simulink model "Ball_Estimation_2_1"  (Simulink 8.0)
settings: Solver=ode4  StartTime=0.0  StopTime=inf  FixedStep=sample_time  RelTol=1e-3
InitFcn:
  | sample_time=0.005;%0.004;%0.0025;%0.02;
  | sample_time_Vicon = 0.005;
  | DeltaT = 0.02;
  | g = 9.81;
  | H0 = g%0.3165;
  | 
  | Q6_mass = 0.95;
  | 
  | Q6_Omega_r = 1.5; %for horizon ref
  | Q6_Zeta_r = 0.7; %for horizon ref
  | Q6_Omega_r_h = 2;%for vertical ref
  | Q6_Zeta_r_h = 1; %for vertical ref
  | 
  | 
  | Q6_Omega = 1.5; %for horizon control
  | Q6_Zeta = 0.7; %for horizon control
  | Q6_Omega_h= 2; %for vertical control
  | Q6_Zeta_h = 0.7; %for vertical control
  | 
  | 
  | Q6_acc_max = 5;%horizontal max acc
  | Q6_acc_max_h = 3;%horizontal max acc
  | 
  | omega_circle = 72*pi/180;
  | omega_h = 0.1;%Ascending speed
  | PI = pi;
  | Circle_R = 2.5;
  | MAX_Height = -2;
undefined symbols (not defined in the file or in its folder): DiscIntNeverNeededParam, PosRefSystem, X330_Control
libraries: simulink x2, dspadpt3 x2
(part 1 of 2)
settings Model: Creator=ttcl3  LastModifiedBy=Vicon
settings SolverCC: MaxConsecutiveMinStep=auto
settings DataIOCC: SignalLoggingSaveFormat=ModelDataLogs
settings DebuggingCC: MultiTaskRateTransMsg=warning  FcnCallInpInsideContextMsg=UseLocalSettings
settings SFSimCC: SimParseCustomCode=off
settings CodeAppCC: CustomSymbolStrType=$N$R$M_T
settings GRTTargetCC: CombineOutputUpdateFcns=off  GRTInterface=on

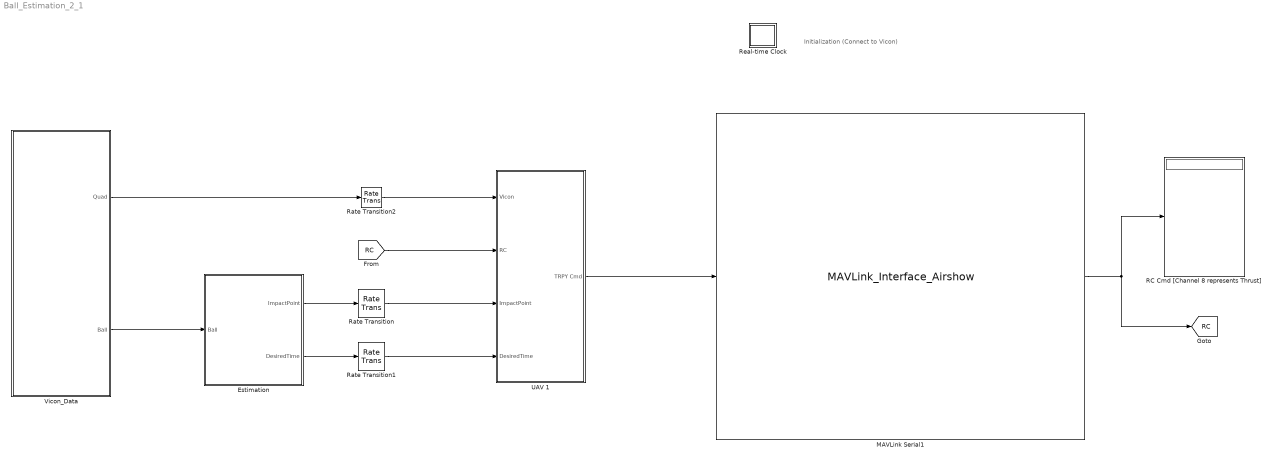
== system Ball_Estimation_2_1 ==
  note: Initialization
      | (Connect to Vicon)
  Estimation : Subsystem
  MAVLink Serial1 : S-Function  FunctionName=MAVLink_Interface_Airshow  Parameters=COM_Port,Baud_Rate,MSG_INPUT,MSG_OUTPUT  EnableBusSupport=off  mask{COM_Port='COM5', Baud_Rate=57600, ATTITUDE_OUT=off, RC_SCALED=on, Quads_1=on, Quads_2=off, Quads_3=off, Quads_4=off, Quads_5=off, Quads_6=off}
      mask prompts: COM_Port "COM Port"; Baud_Rate "Baud Rate"; ATTITUDE_OUT "DEBUG"; RC_SCALED "RC CHANNELS SCALED"; Quads_1 "1 Quad"; Quads_2 "2 Quad"; Quads_3 "3 Quad"; Quads_4 "4 Quad"; Quads_5 "5 Quad"; Quads_6 "6 Quad"
      mask init:
      | MSG_ID_NUM_INPUT = [ uint8(221) uint8(222) uint8(223) uint8(224) uint8(225) uint8(226)];
      | MSG_ID_NAME_INPUT = [Quads_1 Quads_2 Quads_3 Quads_4 Quads_5 Quads_6];
      | 
      | MSG_ID_NUM_OUTPUT = [uint8(34) uint8(30)];
      | MSG_ID_NAME_OUTPUT = [RC_SCALED ATTITUDE_OUT ];
      | 
      | idx_input = find(MSG_ID_NAME_INPUT);
      | MSG_INPUT = MSG_ID_NUM_INPUT(idx_input);
      | 
      | idx_output = find(MSG_ID_NAME_OUTPUT);
      | MSG_OUTPUT = MSG_ID_NUM_OUTPUT(idx_output);
      mask Display:
      | % Block image
      | image(imread('10-inch Quad Heat Map.png'));
      | 
      | %Label block
      | fprintf('MAVLink Serial\n%s\n%dbps', COM_Port,  Baud_Rate)
      | 
      | 
      | %Label input ports
      | 
      | in = 1;
      | if (Quads_1 == 1)
      |     port_label('input', in, 'Quads_1');
      |     in = in + 1;
      | end
      | 
      | if (Quads_2 == 1)
      |     port_label('input', in, 'Quads_2');
      |     in = in + 1;
      | end
      | 
      | if (Quads_3 == 1)
      |     port_label('input', in, 'Quads_3');
      |     in = in + 1;
      | end
      | 
      | if (Quads_4 == 1)
      |     port_label('input', in, 'Quads_4');
      |     in = in + 1;
      | end
      | 
      | if (Quads_5 == 1)
      |     port_label('input', in, 'Quads_5');
      |     in = in + 1;
      | end
      | 
      | 
      | if (Quads_6 == 1)
      |     port_label('input', in, 'Quads_6');
      |     in = in + 1;
      | end
      | %Label output ports
      | 
      | out = 1;
      | if (RC_SCALED == 1)
      |     port_label('output', out, 'RC CMD');
      |     out = out + 1;
      | end
      | 
      | if (ATTITUDE_OUT == 1)
      |     port_label('output', out, 'DEBUG');
      |     out = out + 1;
      | end
  RC Cmd [Channel 8 represents Thrust] : Display
  Rate Transition : RateTransition  OutPortSampleTime=0.02
  Rate Transition1 : RateTransition  OutPortSampleTime=0.02
  Rate Transition2 : RateTransition  OutPortSampleTime=0.02
  Real-time Clock : Subsystem  mask(Real-time Clock){sample_time=0.02, tolerance=1}
      mask prompts: sample_time "Synchronize with real-time every n seconds:"; tolerance "Real-time warning tolerance (seconds):"
      mask help: Real-time Synchronization Block
      mask Help: This block synchronizes simulation time with the PC real-time clock or UNIX system clock. The first dialog entry is the period at which the clock is checked to insure real-time synchronization. The second dialog entry is the number of seconds that the simulation time must be within real-time before a warning is printed.
      mask Display: plot(0,0,100,100,[40,60,60,54,54,64,69,76,82,77,81,83,83,81,78,74,70,64,57,49,41,35,32,30,30,31,34,40,47,47,40,40],[90,90,85,85,80,79,76,87,80,70,64,57,49,41,33,28,24,22,21,23,25,31,37,46,56,65,73,78,80,85,85,90],[69,53,53],[64,50,73])
  UAV 1 : Subsystem
  Vicon_Data : Subsystem
  tag scope: RC=global
  wires:
  Estimation/1(ImpactPoint) -> Rate Transition/1
  Estimation/2(DesiredTime) -> Rate Transition1/1
  [RC] -> UAV 1/2(RC)
  Rate Transition2/1 -> UAV 1/1(Vicon)
  MAVLink Serial1/1 -> [RC], RC Cmd [Channel 8 represents Thrust]/1
  UAV 1/1(TRPY Cmd) -> MAVLink Serial1/1
  Vicon_Data/2(Ball) -> Estimation/1(Ball)
  Vicon_Data/1(Quad) -> Rate Transition2/1
  Rate Transition/1 -> UAV 1/3(ImpactPoint)
  Rate Transition1/1 -> UAV 1/4(DesiredTime)

== system Ball_Estimation_2_1/Estimation ==
  Ball : Inport
  Bus Selector1 : BusSelector  OutputSignals=Position,Velocity
  Trajectory Logic1 : Subsystem
  ImpactPoint : Outport
  DesiredTime : Outport  Port=2
  wires:
  Ball/1 -> Bus Selector1/1
  Bus Selector1/1 -> Trajectory Logic1/1(Ball_Pos)  "<Position>"
  Bus Selector1/2 -> Trajectory Logic1/2(Ball_Vel)  "<Velocity>"
  Trajectory Logic1/1("ImpactPoint ") -> ImpactPoint/1
  Trajectory Logic1/2(DesiredTime) -> DesiredTime/1

== system Ball_Estimation_2_1/Real-time Clock ==
  Real-time Clock : S-Function  FunctionName=rtclock  Parameters=sample_time, tolerance  EnableBusSupport=off

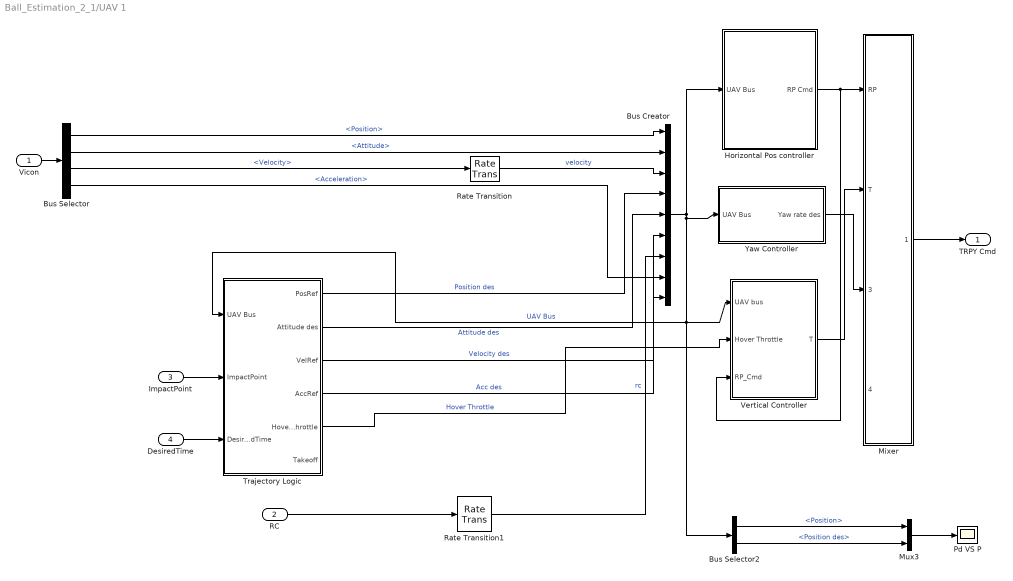
== system Ball_Estimation_2_1/UAV 1 ==
  Vicon : Inport
  RC : Inport  Port=2
  ImpactPoint : Inport  Port=3
  DesiredTime : Inport  Port=4
  Bus Creator : BusCreator  Inputs=9
  Bus Selector : BusSelector  OutputSignals=Position,Attitude,Velocity,Acceleration
  Bus Selector2 : BusSelector  OutputSignals=Position,Position des
  Horizontal Pos controller : Subsystem  AncestorBlock=X330_Control/Horizontal Pos controller  mask{Max_RP=60, Omega=Q6_Omega, PID_i=1, Zeta=Q6_Zeta}
      mask prompts: Max_RP "Cmd Maximum Roll/Pitch (Degree)"; Omega "Omega (P Gain= Omega^2)"; PID_i "I Gain"; Zeta "Zeta (D = 2*Omega*Zeta)"
  Mixer : Subsystem
  Mux3 : Mux  Inputs=2
  Pd VS P : Scope
      settings: TimeRange=19.89708404802744  YMin=-0.75  YMax=0.1
  Rate Transition : RateTransition  OutPortSampleTime=0.02
  Rate Transition1 : RateTransition  OutPortSampleTime=0.02
  Trajectory Logic : Subsystem
  Vertical Controller : Subsystem  AncestorBlock=X330_Control/Vertical Controller  mask{Omega_h=Q6_Omega_h, Zeta_h=Q6_Zeta_h, PID_I_h=1, mass=Q6_mass}
      mask prompts: Omega_h "Omega (P Gain  = Omega^2)"; Zeta_h "Zeta (D Gain = 2*Omega*Zeta)"; PID_I_h "I Gain"
  Yaw Controller : Subsystem  AncestorBlock=X330_Control/Yaw Controller
  TRPY Cmd : Outport
  wires:
  Mux3/1 -> Pd VS P/1
  Bus Selector2/2 -> Mux3/2  "<Position des>"
  Bus Selector2/1 -> Mux3/1  "<Position>"
  Horizontal Pos controller/1(RP Cmd) -> Vertical Controller/3(RP_Cmd), Mixer/1(RP)
  RC/1 -> Rate Transition1/1
  Trajectory Logic/4(AccRef) -> Bus Creator/9  "Acc des"
  Mixer/1(XYZ RPY) -> TRPY Cmd/1
  Vicon/1 -> Bus Selector/1
  Bus Selector/3 -> Rate Transition/1  "<Velocity>"
  Bus Selector/2 -> Bus Creator/2  "<Attitude>"
  Bus Selector/1 -> Bus Creator/1  "<Position>"
  Trajectory Logic/5(HoverThrottle) -> Vertical Controller/2(Hover Throttle)  "Hover Throttle"
  Trajectory Logic/3(VelRef) -> Bus Creator/6  "Velocity des"
  Trajectory Logic/2(Attitude des) -> Bus Creator/5  "Attitude des"
  Trajectory Logic/1(PosRef) -> Bus Creator/4  "Position des"
  Bus Selector/4 -> Bus Creator/8  "<Acceleration>"
  Vertical Controller/1(T) -> Mixer/2(T)
  Yaw Controller/1(Yaw rate des) -> Mixer/3(Yaw rate)
  Bus Creator/1 -> Yaw Controller/1(UAV Bus), Bus Selector2/1, Vertical Controller/1(UAV bus), Trajectory Logic/1(UAV Bus), Horizontal Pos controller/1(UAV Bus)  "UAV Bus"
  Rate Transition1/1 -> Bus Creator/7  "rc"
  Rate Transition/1 -> Bus Creator/3  "velocity"
  ImpactPoint/1 -> Trajectory Logic/2(ImpactPoint)
  DesiredTime/1 -> Trajectory Logic/3(DesiredTime)

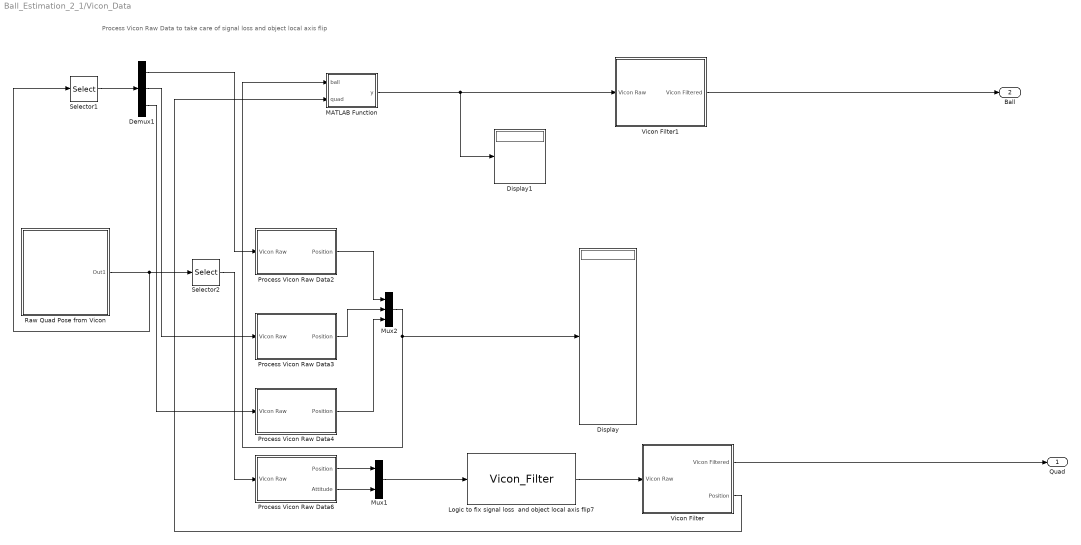
== system Ball_Estimation_2_1/Vicon_Data ==
  note: Process Vicon Raw Data to take care of signal loss and object local axis flip
  Demux1 : Demux  Outputs=3
  Display : Display
  Display1 : Display
  Logic to fix signal loss  and object local axis flip7 : M-S-Function  FunctionName=Vicon_Filter
  MATLAB Function : MATLAB Function  TreatAsAtomicUnit=on
      settings: PermitHierarchicalResolution=ParametersOnly
  Mux1 : Mux  Inputs=2
  Mux2 : Mux  Inputs=3
  Process Vicon Raw Data2 : Subsystem
  Process Vicon Raw Data3 : Subsystem
  Process Vicon Raw Data4 : Subsystem
  Process Vicon Raw Data6 : Subsystem
  Raw Quad Pose from Vicon : Subsystem
  Selector1 : Selector  InputPortWidth=18  IndexOptions=Index vector (dialog)  Indices=[10 11 12 13 14 15 16 17 18]  OutputSizes=1
  Selector2 : Selector  InputPortWidth=18  IndexOptions=Index vector (dialog)  Indices=[1 2 3 4 5 6]  OutputSizes=1
  Vicon Filter : Subsystem  AncestorBlock=X330_Control/Vicon Filter
  Vicon Filter1 : Subsystem  AncestorBlock=X330_Control/Vicon Filter
  Quad : Outport
  Ball : Outport  Port=2
  wires:
  Raw Quad Pose from Vicon/1(Out1) -> Selector1/1, Selector2/1
  Selector2/1 -> Process Vicon Raw Data6/1(Vicon Raw)
  Logic to fix signal loss  and object local axis flip7/1 -> Vicon Filter/1(Vicon Raw)
  Process Vicon Raw Data6/1(Position) -> Mux1/1
  Process Vicon Raw Data6/2(Attitude) -> Mux1/2
  Mux1/1 -> Logic to fix signal loss  and object local axis flip7/1
  Vicon Filter/1(Vicon Filtered) -> Quad/1
  Vicon Filter/2(Position) -> MATLAB Function/2(quad)
  Selector1/1 -> Demux1/1
  Demux1/1 -> Process Vicon Raw Data2/1(Vicon Raw)
  Demux1/2 -> Process Vicon Raw Data3/1(Vicon Raw)
  Demux1/3 -> Process Vicon Raw Data4/1(Vicon Raw)
  Process Vicon Raw Data2/1(Position) -> Mux2/1
  Process Vicon Raw Data3/1(Position) -> Mux2/2
  Process Vicon Raw Data4/1(Position) -> Mux2/3
  Mux2/1 -> MATLAB Function/1(ball), Display/1
  MATLAB Function/1(y) -> Display1/1, Vicon Filter1/1(Vicon Raw)
  Vicon Filter1/1(Vicon Filtered) -> Ball/1

== system Ball_Estimation_2_1/Estimation/Trajectory Logic1 ==
  Ball_Pos : Inport
  Ball_Vel : Inport  Port=2
  Ball pos : Scope
      settings: YMin=-4  YMax=0  SaveName=ScopeData4  MaxDataPoints=50000
  UAV SF : Stateflow chart  TreatAsAtomicUnit=on
      settings: PermitHierarchicalResolution=ParametersOnly
  "ImpactPoint " : Outport
  DesiredTime : Outport  Port=2
  wires:
  Ball_Pos/1 -> Ball pos/1, UAV SF/1(Sc_Pos)
  Ball_Vel/1 -> UAV SF/2(Sc_Vel)
  UAV SF/1(ImpactPoint) -> "ImpactPoint "/1
  UAV SF/2(DesiredTime) -> DesiredTime/1

== system Ball_Estimation_2_1/UAV 1/Horizontal Pos controller ==
  UAV Bus : Inport
  Horizontal Position Controller : Subsystem
  RP Cmd : Outport
  wires:
  Horizontal Position Controller/1(RP Cmd (Radian)) -> RP Cmd/1
  UAV Bus/1 -> Horizontal Position Controller/1(UAV Bus)

== system Ball_Estimation_2_1/UAV 1/Mixer ==
  note: 7x1 vector (usec, XYZRPY)
  RP : Inport
  T : Inport  Port=2
  Yaw rate : Inport  Port=3
  PWM : Inport  Port=4
  Gain : Gain  Gain=180/pi
  Mode : Constant  SampleTime=0.02
  Mux1 : Mux  Inputs=5
  "[-1, 1]" : Fcn  Expr=u(1)*2-1
  XYZ RPY : Outport
  wires:
  "[-1, 1]"/1 -> Mux1/1
  Gain/1 -> Mux1/2
  PWM/1 -> Mux1/5
  Mode/1 -> Mux1/4
  Yaw rate/1 -> Mux1/3
  RP/1 -> Gain/1
  T/1 -> "[-1, 1]"/1
  Mux1/1 -> XYZ RPY/1

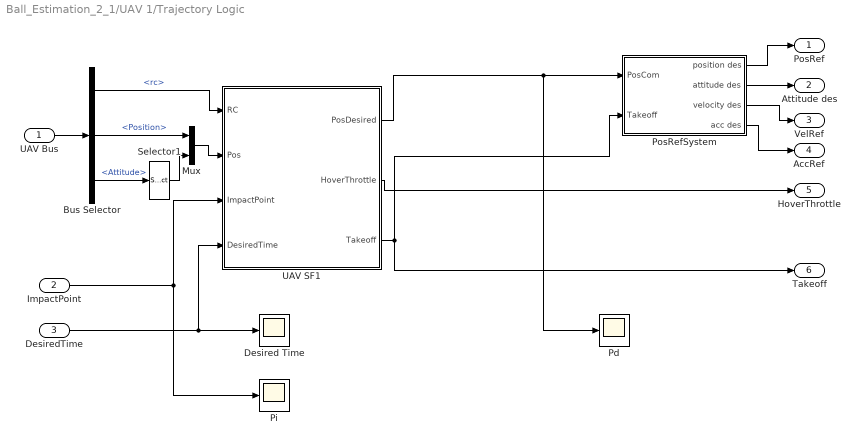
== system Ball_Estimation_2_1/UAV 1/Trajectory Logic ==
  UAV Bus : Inport
  ImpactPoint : Inport  Port=2
  DesiredTime : Inport  Port=3
  Bus Selector : BusSelector  OutputSignals=rc,Position,Attitude
  Desired Time : Scope
      settings: YMin=-0.01  YMax=0.17  SaveName=ScopeData6  MaxDataPoints=500000
  Mux : Mux  Inputs=2
  Pd : Scope
  Pi : Scope
      settings: TimeRange=4.304464104457637  YMin=-0.9662149265126931  YMax=0.8352739072342059  SaveName=ScopeData2
  PosRefSystem : Subsystem  AncestorBlock=X330_Control/PosRefSystem  mask{Omega_r=Q6_Omega_r, Zeta_r=Q6_Zeta_r, Acc_Max=Q6_acc_max, Omega_h_r=Q6_Omega_r_h, Zeta_h_r=Q6_Zeta_r_h, Acc_h_Max=Q6_acc_max_h}
      mask prompts: Omega_r "Omega_r (P Gain= Omega_r^2)"; Zeta_r "Zeta_r (D = 2*Omega_r*Zeta_r)"
  Selector1 : Selector  InputPortWidth=3  IndexOptions=Index vector (dialog)  Indices=[3]  OutputSizes=1
  UAV SF1 : Stateflow chart  TreatAsAtomicUnit=on
      settings: PermitHierarchicalResolution=ParametersOnly
  PosRef : Outport
  Attitude des : Outport  Port=2
  VelRef : Outport  Port=3
  AccRef : Outport  Port=4
  HoverThrottle : Outport  Port=5
  Takeoff : Outport  Port=6
  wires:
  PosRefSystem/2(attitude des) -> Attitude des/1
  PosRefSystem/4(acc des) -> AccRef/1
  PosRefSystem/3(velocity des) -> VelRef/1
  PosRefSystem/1(position des) -> PosRef/1
  Mux/1 -> UAV SF1/2(Pos)
  Selector1/1 -> Mux/2
  Bus Selector/3 -> Selector1/1  "<Attitude>"
  Bus Selector/2 -> Mux/1  "<Position>"
  UAV Bus/1 -> Bus Selector/1
  ImpactPoint/1 -> Pi/1, UAV SF1/3(ImpactPoint)
  UAV SF1/2(HoverThrottle) -> HoverThrottle/1
  Bus Selector/1 -> UAV SF1/1(RC)  "<rc>"
  UAV SF1/3(Takeoff) -> Takeoff/1, PosRefSystem/2(Takeoff)
  DesiredTime/1 -> Desired Time/1, UAV SF1/4(DesiredTime)
  UAV SF1/1(PosDesired) -> Pd/1, PosRefSystem/1(PosCom)

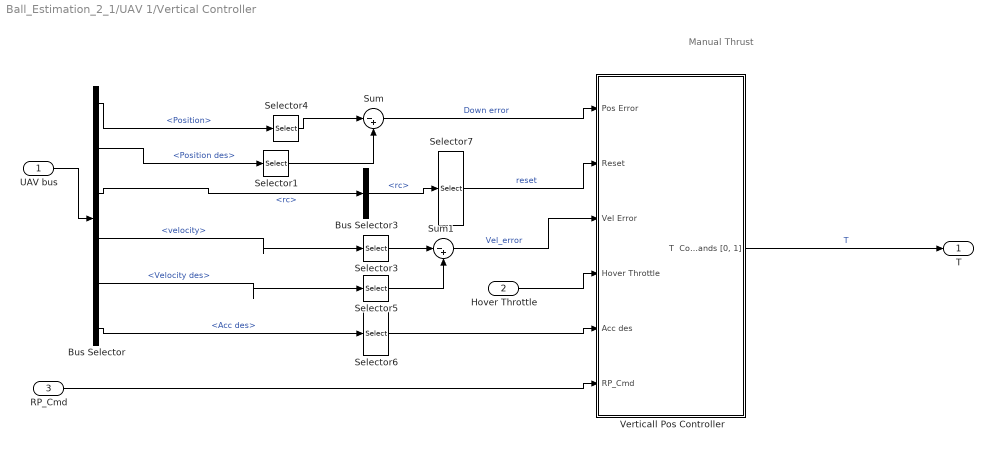
== system Ball_Estimation_2_1/UAV 1/Vertical Controller ==
  note: Manual Thrust
  UAV bus : Inport
  Hover Throttle : Inport  Port=2
  RP_Cmd : Inport  Port=3
  Bus Selector : BusSelector  OutputSignals=Position,Position des,rc,velocity,Velocity des,Acc des
  Bus Selector3 : BusSelector  OutputSignals=rc
  Selector{1,3..5} (4 alike) : Selector  InputPortWidth=3  IndexOptions=Index vector (dialog)  Indices=[3]  OutputSizes=1
  Selector6 : Selector  InputPortWidth=4  IndexOptions=Index vector (dialog)  Indices=[3]  OutputSizes=1
  Selector7 : Selector  InputPortWidth=8  IndexOptions=Index vector (dialog)  Indices=[5]  OutputSizes=1
  Sum : Sum  Inputs=|-+
  Sum1 : Sum  Inputs=|-+
  Verticall Pos Controller : Subsystem
  T : Outport
  wires:
  RP_Cmd/1 -> Verticall Pos Controller/6(RP_Cmd)
  Verticall Pos Controller/1("T  Commands [0, 1]") -> T/1  "T"
  Selector6/1 -> Verticall Pos Controller/5(Acc des)
  Bus Selector/6 -> Selector6/1  "<Acc des>"
  Hover Throttle/1 -> Verticall Pos Controller/4(Hover Throttle)
  Bus Selector/5 -> Selector5/1  "<Velocity des>"
  Bus Selector/4 -> Selector3/1  "<velocity>"
  Selector5/1 -> Sum1/2
  Selector3/1 -> Sum1/1
  Sum1/1 -> Verticall Pos Controller/3(Vel Error)  "Vel_error"
  Selector7/1 -> Verticall Pos Controller/2(Reset)  "reset"
  Bus Selector3/1 -> Selector7/1  "<rc>"
  Selector1/1 -> Sum/2
  Selector4/1 -> Sum/1
  Sum/1 -> Verticall Pos Controller/1(Pos Error)  "Down error"
  Bus Selector/2 -> Selector1/1  "<Position des>"
  Bus Selector/1 -> Selector4/1  "<Position>"
  Bus Selector/3 -> Bus Selector3/1  "<rc>"
  UAV bus/1 -> Bus Selector/1

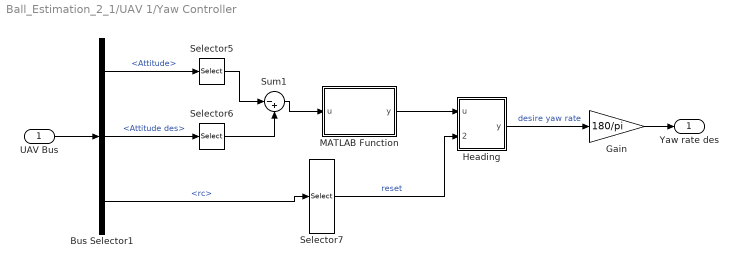
== system Ball_Estimation_2_1/UAV 1/Yaw Controller ==
  UAV Bus : Inport
  Bus Selector1 : BusSelector  OutputSignals=Attitude,Attitude des,rc
  Gain : Gain  Gain=180/pi
  Heading : Subsystem  AncestorBlock=simulink/Continuous/PID Controller  DialogController=pidpack.PIDConfig.pidDDGCreate  DialogControllerArgs=DataTag0  mask(PID 1dof){Controller=PI, TimeDomain=Discrete-time, SampleTime=0.02, IntegratorMethod=Trapezoidal, FilterMethod=Trapezoidal, Form=Parallel, P=3, I=1, D=0, N=100, InitialConditionSource=internal, InitialConditionForIntegrator=0, InitialConditionForFilter=0, ExternalReset=rising, IgnoreLimit=off, ZeroCross=on, LimitOutput=on, UpperSaturationLimit=300*pi/180, LowerSaturationLimit=-300*pi/180, LinearizeAsGain=off, AntiWindupMode=none, Kb=1, TrackingMode=off, Kt=1, RndMeth=Floor, SaturateOnIntegerOverflow=off, LockScale=off, PParamMin=[], PParamMax=[], PParamDataTypeStr=Inherit: Inherit via internal rule, IParamMin=[], IParamMax=[], IParamDataTypeStr=Inherit: Inherit via internal rule, DParamMin=[], DParamMax=[], DParamDataTypeStr=Inherit: Inherit via internal rule, NParamMin=[], NParamMax=[], NParamDataTypeStr=Inherit: Inherit via internal rule, KbParamMin=[], KbParamMax=[], KbParamDataTypeStr=Inherit: Inherit via internal rule, KtParamMin=[], KtParamMax=[], KtParamDataTypeStr=Inherit: Inherit via internal rule, POutMin=[], POutMax=[], POutDataTypeStr=Inherit: Inherit via internal rule, IOutMin=[], IOutMax=[], IOutDataTypeStr=Inherit: Inherit via internal rule, DOutMin=[], DOutMax=[], DOutDataTypeStr=Inherit: Inherit via internal rule, NOutMin=[], NOutMax=[], NOutDataTypeStr=Inherit: Inherit via internal rule, KbOutMin=[], KbOutMax=[], KbOutDataTypeStr=Inherit: Inherit via internal rule, KtOutMin=[], KtOutMax=[], KtOutDataTypeStr=Inherit: Inherit via internal rule, IntegratorOutMin=[], IntegratorOutMax=[], IntegratorOutDataTypeStr=Inherit: Inherit via internal rule, FilterOutMin=[], FilterOutMax=[], FilterOutDataTypeStr=Inherit: Inherit via internal rule, SumOutMin=[], SumOutMax=[], SumOutDataTypeStr=Inherit: Inherit via internal rule, SumI1OutMin=[], SumI1OutMax=[], SumI1OutDataTypeStr=Inherit: Inherit via internal rule, SumI2OutMin=[], SumI2OutMax=[], SumI2OutDataTypeStr=Inherit: Inherit via internal rule, SumI3OutMin=[], SumI3OutMax=[], SumI3OutDataTypeStr=Inherit: Inherit via internal rule, SumDOutMin=[], SumDOutMax=[], SumDOutDataTypeStr=Inherit: Inherit via internal rule, SumAccumDataTypeStr=Inherit: Inherit via internal rule, SumI1AccumDataTypeStr=Inherit: Inherit via internal rule, SumI2AccumDataTypeStr=Inherit: Inherit via internal rule, SumI3AccumDataTypeStr=Inherit: Inherit via internal rule, SumDAccumDataTypeStr=Inherit: Inherit via internal rule, SaturationOutMin=[], SaturationOutMax=[], SaturationOutDataTypeStr=Inherit: Same as input, IntegratorContinuousStateAttributes='', IntegratorStateIdentifier=, IntegratorStateMustResolveToSignalObject=off, IntegratorRTWStateStorageClass=Auto, IntegratorRTWStateStorageTypeQualifier=, FilterContinuousStateAttributes='', FilterStateIdentifier=, FilterStateMustResolveToSignalObject=off, FilterRTWStateStorageClass=Auto, FilterRTWStateStorageTypeQualifier=}
      mask prompts: TimeDomain "Time domain:"; SampleTime "Sample time (-1 for inherited):"; IntegratorMethod "Integrator method:"; FilterMethod "Filter method:"; P "Proportional (P):"; I "Integral (I):"; D "Derivative (D):"; N "Filter coefficient (N):"; InitialConditionSource "Source:"; InitialConditionForIntegrator "Integrator:"; InitialConditionForFilter "Filter:"; ExternalReset "External reset:"; IgnoreLimit "Ignore reset when linearizing"; ZeroCross "Enable zero-crossing detection"; LimitOutput "Limit output"; UpperSaturationLimit "Upper saturation limit:"; LowerSaturationLimit "Lower saturation limit:"; LinearizeAsGain "Ignore saturation when linearizing"; AntiWindupMode "Anti-windup method:"; Kb "Back-calculation coefficient (Kb):"; TrackingMode "Enable tracking mode"; Kt "Tracking coefficient (Kt):"; RndMeth "Integer rounding mode:"; SaturateOnIntegerOverflow "Saturate on integer overflow"; LockScale "Lock data type settings against changes by the fixed-point tools"; PParamMin "P parameter minimum:"; PParamMax "P parameter maximum:"; PParamDataTypeStr "P parameter:"; IParamMin "I parameter minimum:"; IParamMax "I parameter maximum:"; IParamDataTypeStr "I parameter:"; DParamMin "D parameter minimum:"; DParamMax "D parameter maximum:"; DParamDataTypeStr "D parameter:"; NParamMin "N parameter minimum:"; NParamMax "N parameter maximum:"; NParamDataTypeStr "N parameter:"; KbParamMin "Kb parameter minimum:"; KbParamMax "Kb parameter maximum:"; KbParamDataTypeStr "Kb parameter:"; KtParamMin "Kt parameter minimum:"; KtParamMax "Kt parameter maximum:"; KtParamDataTypeStr "Kt parameter:"; POutMin "P product output minimum:"; POutMax "P product output maximum:"; POutDataTypeStr "P product output:"; IOutMin "I product output minimum:"; IOutMax "I product output maximum:"; IOutDataTypeStr "I product output:"; DOutMin "D product output minimum:"; DOutMax "D product output maximum:"; DOutDataTypeStr "D product output:"; NOutMin "N product output minimum:"; NOutMax "N product output maximum:"; NOutDataTypeStr "N product output:"; KbOutMin "Kb product output minimum:"; KbOutMax "Kb product output maximum:"; KbOutDataTypeStr "Kb product output:"; KtOutMin "Kt product output minimum:"; KtOutMax "Kt product output maximum:"; KtOutDataTypeStr "Kt product output:"; IntegratorOutMin "Integrator output minimum:"; IntegratorOutMax "Integrator output maximum:"; IntegratorOutDataTypeStr "Integrator output:"; FilterOutMin "Filter output minimum:"; FilterOutMax "Filter output maximum:"; FilterOutDataTypeStr "Filter output:"; SumOutMin "Sum output minimum:"; SumOutMax "Sum output maximum:"; SumOutDataTypeStr "Sum output:"; SumI1OutMin "SumI1 output minimum:"; SumI1OutMax "SumI1 output maximum:"; SumI1OutDataTypeStr "SumI1 output:"; SumI2OutMin "SumI2 output minimum:"; SumI2OutMax "SumI2 output maximum:"; SumI2OutDataTypeStr "SumI2 output:"; SumI3OutMin "SumI3 output minimum:"; SumI3OutMax "SumI3 output maximum:"; SumI3OutDataTypeStr "SumI3 output:"; SumDOutMin "SumD output minimum:"; SumDOutMax "SumD output maximum:"; SumDOutDataTypeStr "SumD output:"; SumAccumDataTypeStr "Accumulator of Sum:"; SumI1AccumDataTypeStr "Accumulator of SumI1:"; SumI2AccumDataTypeStr "Accumulator of SumI2:"; SumI3AccumDataTypeStr "Accumulator of SumI3:"; SumDAccumDataTypeStr "Accumulator of SumD:"; SaturationOutMin "Saturation output minimum:"; SaturationOutMax "Saturation output maximum:"; SaturationOutDataTypeStr "Saturation output:"; IntegratorContinuousStateAttributes "State name: (e.g., 'position')"; IntegratorStateIdentifier "State name:"; IntegratorStateMustResolveToSignalObject "State name must resolve to Simulink signal object"; IntegratorRTWStateStorageClass "Code generation storage class:"; IntegratorRTWStateStorageTypeQualifier "Code generation storage type qualifier:"; FilterContinuousStateAttributes "State name: (e.g., 'position')"; FilterStateIdentifier "State name:"; FilterStateMustResolveToSignalObject "State name must resolve to Simulink signal object"; FilterRTWStateStorageClass "Code generation storage class:"; FilterRTWStateStorageTypeQualifier "Code generation storage type qualifier:"
      mask help: This block implements continuous- and discrete-time PID control algorithms and includes advanced features such as anti-windup, external reset, and signal tracking. You can tune the PID gains automatically using the 'Tune...' button (requires Simulink Control Design).
      mask init:
      | pidpack.PIDConfig.configPID(gcbh);
      settings: DeleteFcn=pidpack.PIDConfig.closeTuner(gcbh)  ModelCloseFcn=pidpack.PIDConfig.closeTuner(gcbh)  NameChangeFcn=pidpack.PIDConfig.updateTunerName(gcbh)
      mask TypeOptions Controller: PID | PI | PD | P | I
      mask TypeOptions TimeDomain: Continuous-time | Discrete-time
      mask TypeOptions IntegratorMethod: Forward Euler | Backward Euler | Trapezoidal
      mask TypeOptions FilterMethod: Forward Euler | Backward Euler | Trapezoidal
      mask TypeOptions Form: Ideal | Parallel
      mask TypeOptions InitialConditionSource: internal | external
      mask TypeOptions ExternalReset: none | rising | falling | either | level
      mask TypeOptions AntiWindupMode: none | back-calculation | clamping
      mask TypeOptions RndMeth: Ceiling | Convergent | Floor | Nearest | Round | Simplest | Zero
      mask TypeOptions IntegratorRTWStateStorageClass: Auto | ExportedGlobal | ImportedExtern | ImportedExternPointer
      mask TypeOptions FilterRTWStateStorageClass: Auto | ExportedGlobal | ImportedExtern | ImportedExternPointer
      mask Display:
      | image(imread(fullfile(matlabroot,'toolbox','simulink','blocks','@pidpack','@PIDMasks','images','blank.png'),'png'),[0 0 1 1]);
      | disp('PI(z)')
      | port_label('input',1, '');
      | port_label('output',1, '');
      | plot([0 4 4 7]+2,[0 0 8 8]+8);
      | plot([1 4 6]+2,[3 6 3]+8);
      | plot([0 4 6 10]+32,[0 0 8 8]+18);
  MATLAB Function : MATLAB Function  TreatAsAtomicUnit=on
      settings: PermitHierarchicalResolution=ParametersOnly
  Selector5 : Selector  InputPortWidth=3  IndexOptions=Index vector (dialog)  Indices=[3]  OutputSizes=1
  Selector6 : Selector  InputPortWidth=3  IndexOptions=Index vector (dialog)  Indices=[3]  OutputSizes=1
  Selector7 : Selector  InputPortWidth=8  IndexOptions=Index vector (dialog)  Indices=[5]  OutputSizes=1
  Sum1 : Sum  Inputs=|-+
  Yaw rate des : Outport
  wires:
  Bus Selector1/3 -> Selector7/1  "<rc>"
  Bus Selector1/2 -> Selector6/1  "<Attitude des>"
  Selector6/1 -> Sum1/2
  Sum1/1 -> MATLAB Function/1(u)
  MATLAB Function/1(y) -> Heading/1(u)
  UAV Bus/1 -> Bus Selector1/1
  Bus Selector1/1 -> Selector5/1  "<Attitude>"
  Heading/1(y) -> Gain/1  "desire yaw rate"
  Selector7/1 -> Heading/2(RESET)  "reset"
  Selector5/1 -> Sum1/1
  Gain/1 -> Yaw rate des/1

== system Ball_Estimation_2_1/Vicon_Data/Process Vicon Raw Data2 ==
  note: X
  note: Y
  note: Z
  Vicon Raw : Inport
  Demux : Demux  Outputs=3
  Gain1 : Gain  Gain=0.001
  Gain6 : Gain  Gain=-0.001
  Gain7 : Gain  Gain=-0.001
  Matrix Concatenate13 : Concatenate  NumInputs=3  Mode=Multidimensional array
  Position : Outport
  wires:
  Gain1/1 -> Matrix Concatenate13/1
  Demux/1 -> Gain1/1
  Demux/2 -> Gain6/1
  Demux/3 -> Gain7/1
  Gain6/1 -> Matrix Concatenate13/2
  Gain7/1 -> Matrix Concatenate13/3
  Matrix Concatenate13/1 -> Position/1
  Vicon Raw/1 -> Demux/1

== system Ball_Estimation_2_1/Vicon_Data/Process Vicon Raw Data3 ==
  note: Z
  note: Y
  note: X
  Vicon Raw : Inport
  Demux : Demux  Outputs=3
  Gain1 : Gain  Gain=0.001
  Gain6 : Gain  Gain=-0.001
  Gain7 : Gain  Gain=-0.001
  Matrix Concatenate13 : Concatenate  NumInputs=3  Mode=Multidimensional array
  Position : Outport
  wires:
  Vicon Raw/1 -> Demux/1
  Matrix Concatenate13/1 -> Position/1
  Gain7/1 -> Matrix Concatenate13/3
  Gain6/1 -> Matrix Concatenate13/2
  Demux/3 -> Gain7/1
  Demux/2 -> Gain6/1
  Demux/1 -> Gain1/1
  Gain1/1 -> Matrix Concatenate13/1

== system Ball_Estimation_2_1/Vicon_Data/Process Vicon Raw Data4 ==
  note: X
  note: Y
  note: Z
  Vicon Raw : Inport
  Demux : Demux  Outputs=3
  Gain1 : Gain  Gain=0.001
  Gain6 : Gain  Gain=-0.001
  Gain7 : Gain  Gain=-0.001
  Matrix Concatenate13 : Concatenate  NumInputs=3  Mode=Multidimensional array
  Position : Outport
  wires:
  Gain1/1 -> Matrix Concatenate13/1
  Demux/1 -> Gain1/1
  Demux/2 -> Gain6/1
  Demux/3 -> Gain7/1
  Gain6/1 -> Matrix Concatenate13/2
  Gain7/1 -> Matrix Concatenate13/3
  Matrix Concatenate13/1 -> Position/1
  Vicon Raw/1 -> Demux/1

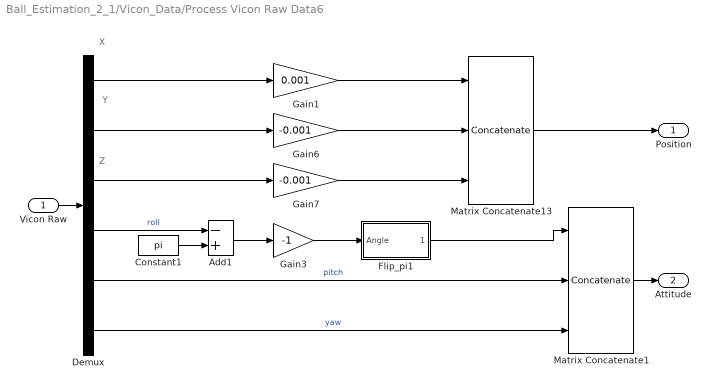
== system Ball_Estimation_2_1/Vicon_Data/Process Vicon Raw Data6 ==
  note: X
  note: Y
  note: Z
  Vicon Raw : Inport
  Add1 : Sum  Inputs=-+
  Constant1 : Constant  Value=pi  OutDataTypeStr=double
  Demux : Demux  Outputs=6
  Flip_pi1 : Subsystem  mask(Flip -pi to pi){}
      mask help: Flips the inputs into the range -pi to pi
      mask Help: Flips the inputs into the range -pi to pi
      mask Display: disp('Flip_pi')
  Gain1 : Gain  Gain=0.001
  Gain3 : Gain  Gain=-1
  Gain6 : Gain  Gain=-0.001
  Gain7 : Gain  Gain=-0.001
  Matrix Concatenate1 : Concatenate  NumInputs=3  Mode=Multidimensional array
  Matrix Concatenate13 : Concatenate  NumInputs=3  Mode=Multidimensional array
  Position : Outport
  Attitude : Outport  Port=2
  wires:
  Constant1/1 -> Add1/2
  Demux/6 -> Matrix Concatenate1/3  "yaw"
  Gain1/1 -> Matrix Concatenate13/1
  Demux/1 -> Gain1/1
  Demux/2 -> Gain6/1
  Demux/3 -> Gain7/1
  Demux/4 -> Add1/1  "roll"
  Gain6/1 -> Matrix Concatenate13/2
  Gain7/1 -> Matrix Concatenate13/3
  Add1/1 -> Gain3/1
  Gain3/1 -> Flip_pi1/1(Angle)
  Demux/5 -> Matrix Concatenate1/2  "pitch"
  Flip_pi1/1(Angle_Flip) -> Matrix Concatenate1/1
  Matrix Concatenate13/1 -> Position/1
  Vicon Raw/1 -> Demux/1
  Matrix Concatenate1/1 -> Attitude/1

== system Ball_Estimation_2_1/Vicon_Data/Raw Quad Pose from Vicon ==
  Constant : Constant
  Interpreted MATLAB Function : MATLABFcn  MATLABFcn=GetViconPose_BallCatching  OutputDimensions=18  SampleTime=0.005
  Out1 : Outport
  wires:
  Constant/1 -> Interpreted MATLAB Function/1
  Interpreted MATLAB Function/1 -> Out1/1

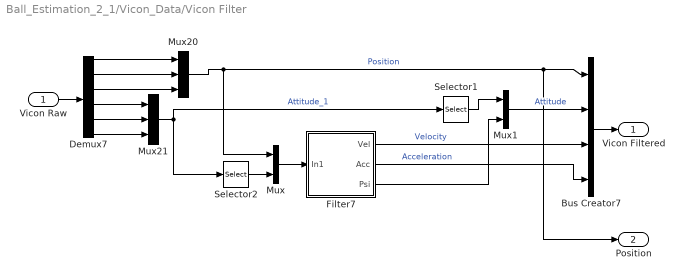
== system Ball_Estimation_2_1/Vicon_Data/Vicon Filter ==
  Vicon Raw : Inport
  Bus Creator7 : BusCreator
  Demux7 : Demux  Outputs=6
  Filter7 : Subsystem
  Mux : Mux  Inputs=2
  Mux1 : Mux  Inputs=2
  Mux20 : Mux  Inputs=3
  Mux21 : Mux  Inputs=3
  Selector1 : Selector  InputPortWidth=3  IndexOptions=Index vector (dialog)  Indices=[1 2]  OutputSizes=1
  Selector2 : Selector  InputPortWidth=3  IndexOptions=Index vector (dialog)  Indices=[3]  OutputSizes=1
  Vicon Filtered : Outport
  Position : Outport  Port=2
  wires:
  Bus Creator7/1 -> Vicon Filtered/1
  Vicon Raw/1 -> Demux7/1
  Mux1/1 -> Bus Creator7/2  "Attitude"
  Selector1/1 -> Mux1/1
  Filter7/3(Psi) -> Mux1/2
  Mux/1 -> Filter7/1(In1)
  Selector2/1 -> Mux/2
  Filter7/2(Acc) -> Bus Creator7/4  "Acceleration"
  Filter7/1(Vel) -> Bus Creator7/3  "Velocity"
  Mux21/1 -> Selector1/1, Selector2/1  "Attitude_1"
  Mux20/1 -> Mux/1, Position/1, Bus Creator7/1  "Position"
  Demux7/2 -> Mux20/2
  Demux7/1 -> Mux20/1
  Demux7/6 -> Mux21/3
  Demux7/5 -> Mux21/2
  Demux7/4 -> Mux21/1
  Demux7/3 -> Mux20/3

== system Ball_Estimation_2_1/Vicon_Data/Vicon Filter1 ==
  Vicon Raw : Inport
  Bus Creator7 : BusCreator  Inputs=3
  Demux7 : Demux  Outputs=6
  Filter7 : Subsystem
  Mux : Mux  Inputs=2
  Mux20 : Mux  Inputs=3
  Mux21 : Mux  Inputs=3
  Selector2 : Selector  InputPortWidth=3  IndexOptions=Index vector (dialog)  Indices=[3]  OutputSizes=1
  Vicon Filtered : Outport
  wires:
  Demux7/3 -> Mux20/3
  Demux7/4 -> Mux21/1
  Demux7/5 -> Mux21/2
  Demux7/6 -> Mux21/3
  Demux7/1 -> Mux20/1
  Demux7/2 -> Mux20/2
  Mux20/1 -> Bus Creator7/1, Mux/1  "Position"
  Mux21/1 -> Selector2/1  "Attitude_1"
  Filter7/1(Vel) -> Bus Creator7/2  "Velocity"
  Filter7/2(Acc) -> Bus Creator7/3  "Acceleration"
  Selector2/1 -> Mux/2
  Mux/1 -> Filter7/1(In1)
  Vicon Raw/1 -> Demux7/1
  Bus Creator7/1 -> Vicon Filtered/1

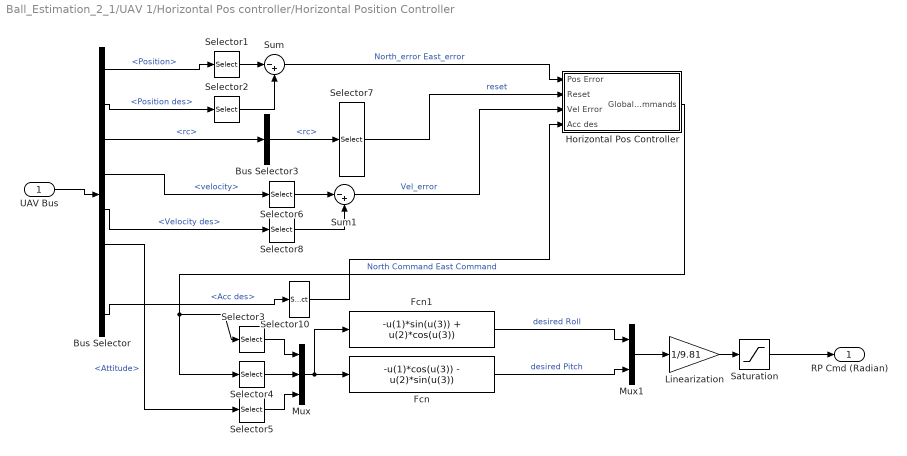
== system Ball_Estimation_2_1/UAV 1/Horizontal Pos controller/Horizontal Position Controller ==
  UAV Bus : Inport
  Bus Selector : BusSelector  OutputSignals=Position,Position des,rc,velocity,Velocity des,Attitude,Acceleration,Acc des
  Bus Selector3 : BusSelector  OutputSignals=rc
  Fcn : Fcn  Expr=-u(1)*cos(u(3)) - u(2)*sin(u(3))
  Fcn1 : Fcn  Expr=-u(1)*sin(u(3)) + u(2)*cos(u(3))
  Horizontal Pos Controller : Subsystem
  Linearization : Gain  Gain=1/9.81  OutDataTypeStr=double
  Mux : Mux  Inputs=3
  Mux1 : Mux  Inputs=2
  Saturation : Saturate  UpperLimit=Max_RP  LowerLimit=-Max_RP
  Selector{1..2,6,8} (4 alike) : Selector  InputPortWidth=3  IndexOptions=Index vector (dialog)  Indices=[1 2]  OutputSizes=1
  Selector10 : Selector  InputPortWidth=4  IndexOptions=Index vector (dialog)  Indices=[1 2]  OutputSizes=1
  Selector3 : Selector  InputPortWidth=2  IndexOptions=Index vector (dialog)  Indices=[1]  OutputSizes=1
  Selector4 : Selector  InputPortWidth=2  IndexOptions=Index vector (dialog)  Indices=[2]  OutputSizes=1
  Selector5 : Selector  InputPortWidth=3  IndexOptions=Index vector (dialog)  Indices=[3]  OutputSizes=1
  Selector7 : Selector  InputPortWidth=8  IndexOptions=Index vector (dialog)  Indices=[5]  OutputSizes=1
  Sum : Sum  Inputs=|-+
  Sum1 : Sum  Inputs=|-+
  RP Cmd (Radian) : Outport
  wires:
  Saturation/1 -> RP Cmd (Radian)/1
  Linearization/1 -> Saturation/1
  Selector10/1 -> Horizontal Pos Controller/4(Acc des)
  Bus Selector/8 -> Selector10/1  "<Acc des>"
  Bus Selector/5 -> Selector8/1  "<Velocity des>"
  Bus Selector/4 -> Selector6/1  "<velocity>"
  Bus Selector/3 -> Bus Selector3/1  "<rc>"
  Selector8/1 -> Sum1/2
  Selector6/1 -> Sum1/1
  Sum1/1 -> Horizontal Pos Controller/3(Vel Error)  "Vel_error"
  Selector7/1 -> Horizontal Pos Controller/2(Reset)  "reset"
  Bus Selector3/1 -> Selector7/1  "<rc>"
  Mux1/1 -> Linearization/1
  Fcn/1 -> Mux1/2  "desired Pitch"
  Fcn1/1 -> Mux1/1  "desired Roll"
  Mux/1 -> Fcn1/1, Fcn/1
  Selector5/1 -> Mux/3
  Selector4/1 -> Mux/2
  Selector3/1 -> Mux/1
  Bus Selector/6 -> Selector5/1  "<Attitude>"
  Horizontal Pos Controller/1(Global Commands) -> Selector4/1, Selector3/1  "North Command East Command"
  UAV Bus/1 -> Bus Selector/1
  Selector2/1 -> Sum/2
  Selector1/1 -> Sum/1
  Bus Selector/2 -> Selector2/1  "<Position des>"
  Bus Selector/1 -> Selector1/1  "<Position>"
  Sum/1 -> Horizontal Pos Controller/1(Pos Error)  "North_error East_error"

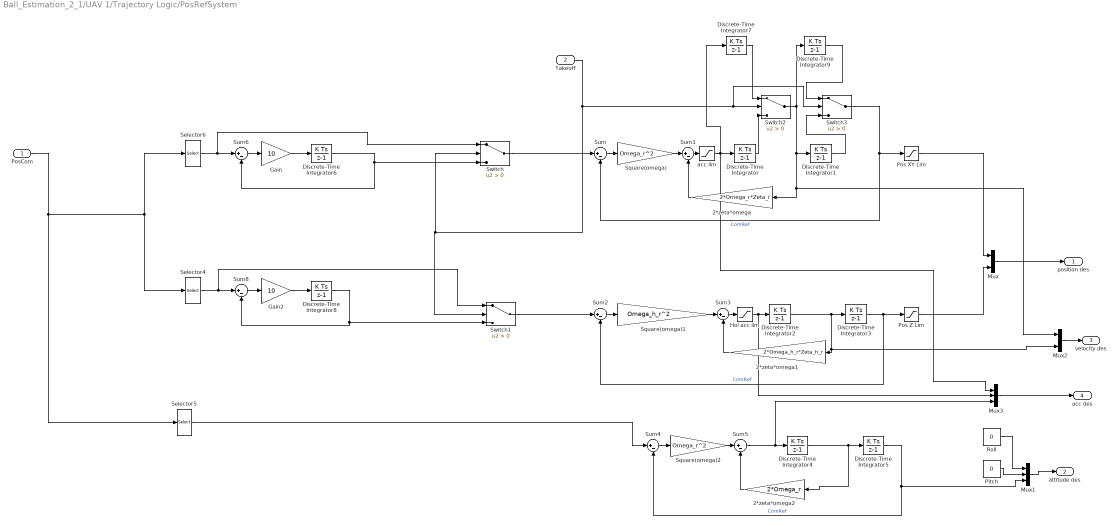
== system Ball_Estimation_2_1/UAV 1/Trajectory Logic/PosRefSystem ==
  PosCom : Inport
  Takeoff : Inport  Port=2
  2*zeta*omega : Gain  Gain=2*Omega_r*Zeta_r
  2*zeta*omega1 : Gain  Gain=2*Omega_h_r*Zeta_h_r
  2*zeta*omega2 : Gain  Gain=2*Omega_r
  Discrete-Time Integrator{,1..2,7,9} (5 alike) : DiscreteIntegrator  gainval=1  SampleTime=-1  ICPrevOutput=DiscIntNeverNeededParam  ICPrevScaledInput=DiscIntNeverNeededParam
  Discrete-Time Integrator{3..6,8} (5 alike) : DiscreteIntegrator  SampleTime=-1  ICPrevOutput=DiscIntNeverNeededParam  ICPrevScaledInput=DiscIntNeverNeededParam
  Gain : Gain  Gain=10
  Gain2 : Gain  Gain=10
  Hol acc lim : Saturate  UpperLimit=Acc_h_Max  LowerLimit=-Acc_h_Max
  Mux : Mux  Inputs=2
  Mux1 : Mux  Inputs=3
  Mux2 : Mux  Inputs=2
  Mux3 : Mux  Inputs=3
  Pitch : Constant  Value=0  SampleTime=0.02
  Pos XY Lim : Saturate  UpperLimit=3  LowerLimit=-3
  Pos Z Lim : Saturate  LowerLimit=-3
  Roll : Constant  Value=0  SampleTime=0.02
  Selector4 : Selector  InputPortWidth=4  IndexOptions=Index vector (dialog)  Indices=[3]  OutputSizes=1
  Selector5 : Selector  InputPortWidth=4  IndexOptions=Index vector (dialog)  Indices=[4]  OutputSizes=1
  Selector6 : Selector  InputPortWidth=4  IndexOptions=Index vector (dialog)  Indices=[1 2]  OutputSizes=1
  Square(omega) : Gain  Gain=Omega_r^2
  Square(omega)1 : Gain  Gain=Omega_h_r^2
  Square(omega)2 : Gain  Gain=Omega_r^2
  Sum{,1..6,8} (8 alike) : Sum  Inputs=|+-
  Switch{,1..3} (4 alike) : Switch  Criteria=u2 > Threshold
  acc lim : Saturate  UpperLimit=Acc_Max  LowerLimit=-Acc_Max
  position des : Outport
  attitude des : Outport  Port=2
  velocity des : Outport  Port=3
  acc des : Outport  Port=4
  wires:
  Pos Z Lim/1 -> Mux/2
  Pos XY Lim/1 -> Mux/1
  Sum8/1 -> Gain2/1
  Gain2/1 -> Discrete-Time Integrator8/1
  Discrete-Time Integrator8/1 -> Switch1/3, Sum8/2
  Sum6/1 -> Gain/1
  Gain/1 -> Discrete-Time Integrator6/1
  Discrete-Time Integrator6/1 -> Switch/3, Sum6/2
  Mux3/1 -> acc des/1
  Mux2/1 -> velocity des/1
  Mux1/1 -> attitude des/1
  Pitch/1 -> Mux1/2
  Roll/1 -> Mux1/1
  Mux/1 -> position des/1
  Switch3/1 -> Pos XY Lim/1, Sum/2  "ComRef"
  Selector5/1 -> Sum4/1
  2*zeta*omega2/1 -> Sum5/2
  Sum5/1 -> Mux3/3, Discrete-Time Integrator4/1
  Discrete-Time Integrator4/1 -> 2*zeta*omega2/1, Discrete-Time Integrator5/1
  Square(omega)2/1 -> Sum5/1
  Sum4/1 -> Square(omega)2/1
  Discrete-Time Integrator5/1 -> Mux1/3, Sum4/2  "ComRef"
  Hol acc lim/1 -> Mux3/2, Discrete-Time Integrator2/1
  2*zeta*omega1/1 -> Sum3/2
  Sum3/1 -> Hol acc lim/1
  Discrete-Time Integrator2/1 -> Mux2/2, 2*zeta*omega1/1, Discrete-Time Integrator3/1
  Square(omega)1/1 -> Sum3/1
  Sum2/1 -> Square(omega)1/1
  Discrete-Time Integrator3/1 -> Pos Z Lim/1, Sum2/2  "ComRef"
  acc lim/1 -> Discrete-Time Integrator7/1, Mux3/1, Discrete-Time Integrator/1
  2*zeta*omega/1 -> Sum1/2
  Sum1/1 -> acc lim/1
  Switch2/1 -> Mux2/1, 2*zeta*omega/1, Discrete-Time Integrator1/1, Discrete-Time Integrator9/1
  Square(omega)/1 -> Sum1/1
  Sum/1 -> Square(omega)/1
  Takeoff/1 -> Switch3/2, Switch2/2, Switch1/2, Switch/2
  PosCom/1 -> Selector4/1, Selector6/1, Selector5/1
  Switch/1 -> Sum/1
  Switch1/1 -> Sum2/1
  Selector6/1 -> Switch/1, Sum6/1
  Selector4/1 -> Switch1/1, Sum8/1
  Discrete-Time Integrator/1 -> Switch2/3
  Discrete-Time Integrator7/1 -> Switch2/1
  Discrete-Time Integrator9/1 -> Switch3/1
  Discrete-Time Integrator1/1 -> Switch3/3

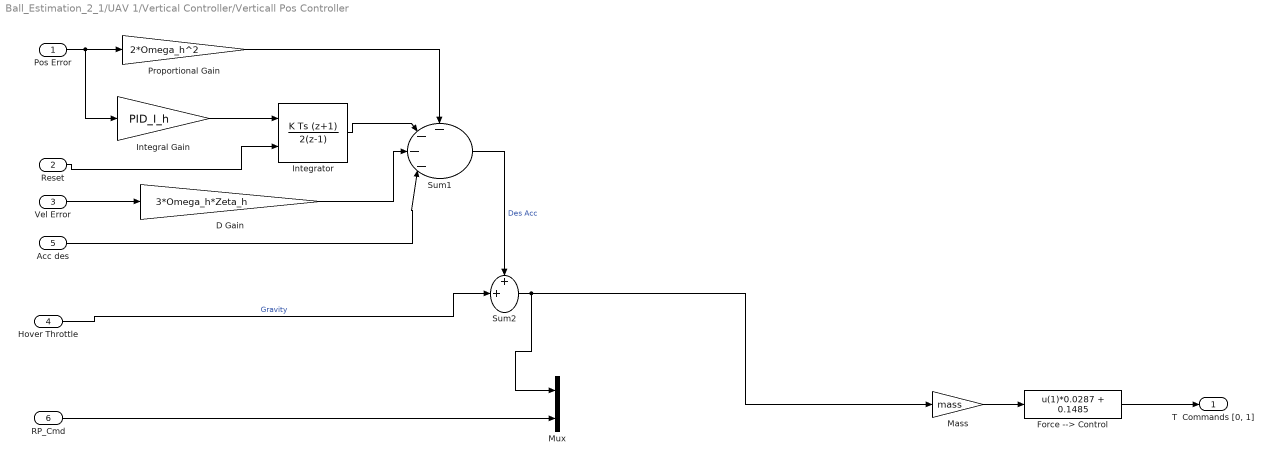
== system Ball_Estimation_2_1/UAV 1/Vertical Controller/Verticall Pos Controller ==
  Pos Error : Inport
  Reset : Inport  Port=2
  Vel Error : Inport  Port=3
  Hover Throttle : Inport  Port=4
  Acc des : Inport  Port=5
  RP_Cmd : Inport  Port=6
  D Gain : Gain  Gain=3*Omega_h*Zeta_h  OutDataTypeStr=double
  Force --> Control : Fcn  Expr=u(1)*0.0287 + 0.1485
  Integral Gain : Gain  DisableCoverage=on  Gain=PID_I_h  ParamDataTypeStr=double  OutDataTypeStr=double
  Integrator : DiscreteIntegrator  DisableCoverage=on  IntegratorMethod=Integration: Trapezoidal  ExternalReset=rising  InitialConditionMode=State only (most efficient)  SampleTime=-1  OutDataTypeStr=double  UpperSaturationLimit=0.3  LowerSaturationLimit=-0.3  ICPrevOutput=DiscIntNeverNeededParam  ICPrevScaledInput=DiscIntNeverNeededParam
  Mass : Gain  DisableCoverage=on  Gain=mass  ParamDataTypeStr=double  OutDataTypeStr=double
  Mux : Mux  Inputs=2
  Proportional Gain : Gain  DisableCoverage=on  Gain=2*Omega_h^2  ParamDataTypeStr=double  OutDataTypeStr=double
  Sum1 : Sum  DisableCoverage=on  Inputs=----|  AccumDataTypeStr=double  OutDataTypeStr=double  SampleTime=0.02
  Sum2 : Sum  DisableCoverage=on  Inputs=++|  AccumDataTypeStr=double  OutDataTypeStr=double  SampleTime=0.02
  "T  Commands [0, 1]" : Outport
  wires:
  Force --> Control/1 -> "T  Commands [0, 1]"/1
  Sum2/1 -> Mass/1, Mux/1
  RP_Cmd/1 -> Mux/2
  Mass/1 -> Force --> Control/1
  Sum1/1 -> Sum2/1  "Des Acc"
  Hover Throttle/1 -> Sum2/2  "Gravity"
  Acc des/1 -> Sum1/4
  D Gain/1 -> Sum1/3
  Vel Error/1 -> D Gain/1
  Reset/1 -> Integrator/2
  Pos Error/1 -> Integral Gain/1, Proportional Gain/1
  Proportional Gain/1 -> Sum1/1
  Integrator/1 -> Sum1/2
  Integral Gain/1 -> Integrator/1

== system Ball_Estimation_2_1/UAV 1/Yaw Controller/Heading ==
  u : Inport  SampleTime=SampleTime
  RESET : Inport  Port=2  SampleTime=SampleTime
  Integral Gain : Gain  DisableCoverage=on  Gain=I  ParamMin=IParamMin  ParamMax=IParamMax  ParamDataTypeStr=IParamDataTypeStr  OutMin=IOutMin  OutMax=IOutMax  OutDataTypeStr=IOutDataTypeStr
  Integrator : DiscreteIntegrator  DisableCoverage=on  IntegratorMethod=Integration: Trapezoidal  ExternalReset=rising  InitialCondition=InitialConditionForIntegrator  InitialConditionMode=State only (most efficient)  SampleTime=-1  OutMin=IntegratorOutMin  OutMax=IntegratorOutMax  OutDataTypeStr=IntegratorOutDataTypeStr  ICPrevOutput=DiscIntNeverNeededParam  ICPrevScaledInput=DiscIntNeverNeededParam
  Proportional Gain : Gain  DisableCoverage=on  Gain=P  ParamMin=PParamMin  ParamMax=PParamMax  ParamDataTypeStr=PParamDataTypeStr  OutMin=POutMin  OutMax=POutMax  OutDataTypeStr=POutDataTypeStr
  Saturation : Saturate  UpperLimit=UpperSaturationLimit  LowerLimit=LowerSaturationLimit  LinearizeAsGain=off  OutMin=SaturationOutMin  OutMax=SaturationOutMax  OutDataTypeStr=SaturationOutDataTypeStr
  Sum : Sum  DisableCoverage=on  Inputs=++|  AccumDataTypeStr=SumAccumDataTypeStr  OutMin=SumOutMin  OutMax=SumOutMax  OutDataTypeStr=SumOutDataTypeStr
  y : Outport  InitialOutput=0
  wires:
  u/1 -> Integral Gain/1, Proportional Gain/1
  Integral Gain/1 -> Integrator/1
  Integrator/1 -> Sum/2
  Proportional Gain/1 -> Sum/1
  RESET/1 -> Integrator/2
  Saturation/1 -> y/1
  Sum/1 -> Saturation/1

== system Ball_Estimation_2_1/Vicon_Data/Process Vicon Raw Data6/Flip_pi1 ==
  Angle : Inport
  Add : Sum  Inputs=-+
  Compare To Constant1 : simulink/Logic and Bit Operations/Compare To Constant  relop=>  const=pi  OutDataTypeStr=uint8  ZeroCross=off
  Constant : Constant  Value=2*pi
  Data Type Duplicate : DataTypeDuplicate
  Flip_0_to_2pi : Subsystem  mask(Flip zero to 2pi){}
      mask help: Flips the inputs into the range zero to +2pi
      mask Help: Flips the inputs into the range zero to +2pi
      mask Display: disp('Flip_0_2pi')
  Switch : Switch  Criteria=u2 ~= 0
  Angle_Flip : Outport
  wires:
  Switch/1 -> Data Type Duplicate/1, Angle_Flip/1
  Add/1 -> Switch/1
  Constant/1 -> Add/1
  Compare To Constant1/1 -> Switch/2
  Flip_0_to_2pi/1(Angle_Flip) -> Add/2, Compare To Constant1/1, Switch/3
  Angle/1 -> Data Type Duplicate/2, Flip_0_to_2pi/1(Angle)

== system Ball_Estimation_2_1/Vicon_Data/Vicon Filter/Filter7 ==
  In1 : Inport
  Kalman Filter : dspadpt3/Kalman Filter  num_targets=1  sourceEnable=Always  isReset=on  X=zeros([12, 1])  P=zeros(12)  A=[1 sample_time_Vicon sample_time_Vicon*sample_time_Vicon/2 zeros(1,9);0 1 sample_time_Vicon zeros(1,9);0 0 1 zeros(1,9);0 0 0 1 sample_time_Vicon sample_time_Vicon*sample_time_Vicon/2 zeros(1,6);zeros(1,4) 1 sample_time_Vicon zeros(1,6);zeros(1,5) 1 zeros(1,6);zeros(1,6) 1 sample_time_Vicon sample_time_Vicon*sample_time_Vicon/2 zeros(1,3);zeros(1,7) 1 sample_time_Vicon zeros(1,3);zeros(1,8) 1 zeros(1,3);zeros(1,9) 1 sample_time_Vicon sample_time_Vicon*sample_time_Vicon/2;zeros(1,10) 1 sample_time_Vicon;zeros(1,11) 1];  sourceMeasure=Specify via Dialog  H=[1 zeros(1,11); zeros(1,3) 1 zeros(1,8);zeros(1,6) 1 zeros(1,5);zeros(1,9) 1 0 0]  Q=diag([0 0.001 0.001 0 0.001 0.001 0 0.001 0.001 0 0.001 0.001]);  R=diag([0.001 0.001 0.001 0.05])  isOutputEstMeasure=off  isOutputEstState=on  isOutputEstError=off  isOutputPrdMeasure=off  isOutputPrdState=off  isOutputPrdError=off
  Selector1 : Selector  InputPortWidth=12  IndexOptions=Index vector (dialog)  Indices=[10]  OutputSizes=1
  Selector5 : Selector  InputPortWidth=12  IndexOptions=Index vector (dialog)  Indices=[2 5 8]  OutputSizes=1
  Selector6 : Selector  InputPortWidth=12  IndexOptions=Index vector (dialog)  Indices=[3 6 9]  OutputSizes=1
  Vel : Outport
  Acc : Outport  Port=2
  Psi : Outport  Port=3
  wires:
  Selector1/1 -> Psi/1
  Selector5/1 -> Vel/1
  In1/1 -> Kalman Filter/1
  Kalman Filter/1 -> Selector1/1, Selector5/1, Selector6/1
  Selector6/1 -> Acc/1

== system Ball_Estimation_2_1/Vicon_Data/Vicon Filter1/Filter7 ==
  In1 : Inport
  Kalman Filter : dspadpt3/Kalman Filter  num_targets=1  sourceEnable=Always  isReset=on  X=zeros([12, 1])  P=zeros(12)  A=[1 sample_time_Vicon sample_time_Vicon*sample_time_Vicon/2 zeros(1,9);0 1 sample_time_Vicon zeros(1,9);0 0 1 zeros(1,9);0 0 0 1 sample_time_Vicon sample_time_Vicon*sample_time_Vicon/2 zeros(1,6);zeros(1,4) 1 sample_time_Vicon zeros(1,6);zeros(1,5) 1 zeros(1,6);zeros(1,6) 1 sample_time_Vicon sample_time_Vicon*sample_time_Vicon/2 zeros(1,3);zeros(1,7) 1 sample_time_Vicon zeros(1,3);zeros(1,8) 1 zeros(1,3);zeros(1,9) 1 sample_time_Vicon sample_time_Vicon*sample_time_Vicon/2;zeros(1,10) 1 sample_time_Vicon;zeros(1,11) 1];  sourceMeasure=Specify via Dialog  H=[1 zeros(1,11); zeros(1,3) 1 zeros(1,8);zeros(1,6) 1 zeros(1,5);zeros(1,9) 1 0 0]  Q=diag([0 0.001 0.001 0 0.001 0.001 0 0.001 0.001 0 0.001 0.001]);  R=diag([0.001 0.001 0.001 0.05])  isOutputEstMeasure=off  isOutputEstState=on  isOutputEstError=off  isOutputPrdMeasure=off  isOutputPrdState=off  isOutputPrdError=off
  Selector5 : Selector  InputPortWidth=12  IndexOptions=Index vector (dialog)  Indices=[2 5 8]  OutputSizes=1
  Selector6 : Selector  InputPortWidth=12  IndexOptions=Index vector (dialog)  Indices=[3 6 9]  OutputSizes=1
  Vel : Outport
  Acc : Outport  Port=2
  wires:
  Selector6/1 -> Acc/1
  Kalman Filter/1 -> Selector6/1, Selector5/1
  In1/1 -> Kalman Filter/1
  Selector5/1 -> Vel/1

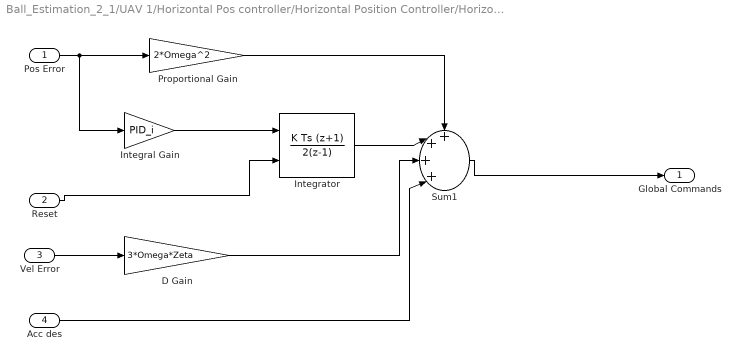
== system Ball_Estimation_2_1/UAV 1/Horizontal Pos controller/Horizontal Position Controller/Horizontal Pos Controller ==
  Pos Error : Inport
  Reset : Inport  Port=2
  Vel Error : Inport  Port=3
  Acc des : Inport  Port=4
  D Gain : Gain  Gain=3*Omega*Zeta  OutDataTypeStr=double
  Integral Gain : Gain  DisableCoverage=on  Gain=PID_i  ParamDataTypeStr=double  OutDataTypeStr=double
  Integrator : DiscreteIntegrator  DisableCoverage=on  IntegratorMethod=Integration: Trapezoidal  ExternalReset=rising  InitialConditionMode=State only (most efficient)  SampleTime=-1  OutDataTypeStr=double  UpperSaturationLimit=10*pi/180  LowerSaturationLimit=-10*pi/180  ICPrevOutput=DiscIntNeverNeededParam  ICPrevScaledInput=DiscIntNeverNeededParam
  Proportional Gain : Gain  DisableCoverage=on  Gain=2*Omega^2  ParamDataTypeStr=double  OutDataTypeStr=double
  Sum1 : Sum  DisableCoverage=on  Inputs=++++|  AccumDataTypeStr=double  OutDataTypeStr=double  SampleTime=0.02
  Global Commands : Outport
  wires:
  Acc des/1 -> Sum1/4
  D Gain/1 -> Sum1/3
  Vel Error/1 -> D Gain/1
  Reset/1 -> Integrator/2
  Pos Error/1 -> Integral Gain/1, Proportional Gain/1
  Sum1/1 -> Global Commands/1
  Proportional Gain/1 -> Sum1/1
  Integrator/1 -> Sum1/2
  Integral Gain/1 -> Integrator/1

== system Ball_Estimation_2_1/Vicon_Data/Process Vicon Raw Data6/Flip_pi1/Flip_0_to_2pi ==
  Angle : Inport
  Add : Sum
  Compare To Constant1 : simulink/Logic and Bit Operations/Compare To Constant  relop=<  const=0  OutDataTypeStr=uint8  ZeroCross=off
  Constant : Constant  Value=2*pi
  Data Type Duplicate : DataTypeDuplicate
  Flip_2pi : Subsystem  mask(Flip -2pi to 2pi){}
      mask help: Flips the inputs into the range -2pi to +2pi
      mask Help: Flips the inputs into the range -2pi to +2pi
      mask Display: disp('Flip_2pi')
  Switch : Switch  Criteria=u2 ~= 0
  Angle_Flip : Outport
  wires:
  Switch/1 -> Data Type Duplicate/1, Angle_Flip/1
  Angle/1 -> Data Type Duplicate/2, Flip_2pi/1(Angle)
  Add/1 -> Switch/1
  Constant/1 -> Add/1
  Compare To Constant1/1 -> Switch/2
  Flip_2pi/1(Angle_Flip) -> Switch/3, Add/2, Compare To Constant1/1

== system Ball_Estimation_2_1/Vicon_Data/Process Vicon Raw Data6/Flip_pi1/Flip_0_to_2pi/Flip_2pi ==
  Angle : Inport
  Bias : Bias  Bias=-2*pi
  Constant : Constant  Value=2*pi
  Data Type Duplicate : DataTypeDuplicate
  Modulo : Math  Operator=mod  SaturateOnIntegerOverflow=on
  Sign1 : Signum
  Switch : Switch
  Angle_Flip : Outport
  wires:
  Switch/1 -> Data Type Duplicate/2, Angle_Flip/1
  Bias/1 -> Switch/3
  Sign1/1 -> Switch/2
  Modulo/1 -> Switch/1, Bias/1
  Constant/1 -> Modulo/2
  Angle/1 -> Data Type Duplicate/1, Sign1/1, Modulo/1

== matlab function Vicon_Data/MATLAB Function ==
  data: ball input double; y output double; quad input double
function y = fcn(ball, quad)
%#codegen
ball1 = ball;
temp = zeros(3,1);

count = 0;
xmin = -4;
xmax = 4;
ymin = -2;
ymax = 1;
zmin = -2.5;
zmax = -0.05;
for i=0:2;
    %eliminate noise from outside and the quad
    if(norm(ball1(3*i+1:3*i+3)-quad,2) < 0.1)
        ball1(3*i+1:3*i+3) = zeros(3,1);
    end;
    if((ball1(3*i+1)>xmax)||(ball1(3*i+1)<xmin)||(ball1(3*i+2)>ymax)||(ball1(3*i+2)<ymin)||(ball1(3*i+3)>zmax)||(ball1(3*i+3)<zmin))
        ball1(3*i+1:3*i+3) = zeros(3,1);
    end;
    if(ball1(3*i+1)~=0)||(ball1(3*i+2)~=0)
        count = count + 1;
        temp = temp + ball1(3*i+1:3*i+3);
    end;
end;

y = zeros(6,1);
if(count == 1)    
    y(1) = temp(1);
    y(2) = temp(2);
    y(3) = temp(3);
end;

end
